simulink subsystem "CLAW_for_QGC_Mission"  (R2024a)
settings: Solver=VariableStepAuto  StartTime=0.0  StopTime=10.0  RelTol=1e-3
undefined symbols (not defined in the file or in its folder): MC_PITCH_P, MC_PITCHRATE_D, MC_PITCHRATE_I, MC_PITCHRATE_P, MC_ROLL_P, MC_ROLLRATE_D, MC_ROLLRATE_I, MC_ROLLRATE_P, MC_YAW_P, MC_YAWRATE_D, MC_YAWRATE_I, MC_YAWRATE_P, MPC_XY_P, MPC_XY_VEL_MAX, MPC_Z_D, MPC_Z_I, MPC_Z_P, MPC_Z_VEL_D_ACC, MPC_Z_VEL_I_ACC, MPC_Z_VEL_MAX_DN, MPC_Z_VEL_MAX_UP, MPC_Z_VEL_P_ACC, pitch, pitch_body, roll, roll_body, thrust_body, timestamp, yaw, yaw_body
libraries: px4lib x25, slpidlib x10, px4uORBlib x4, simulink_extras x4, px4Utilslib x2, sharedutil x1, sharedtransform x1, simulink x1
(part 1 of 2)
settings Model: Creator=user  LastModifiedBy=user

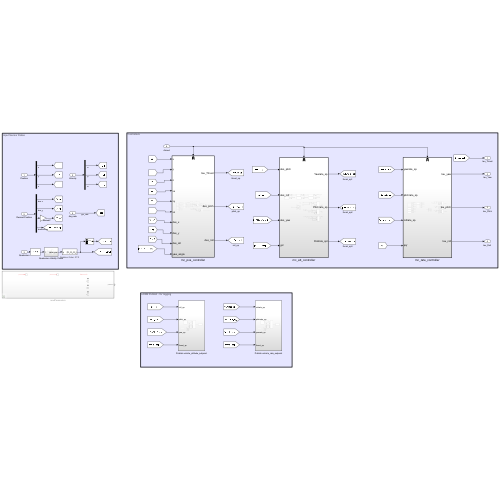
[thumbnail: Simulink's stored preview of the top-level diagram]
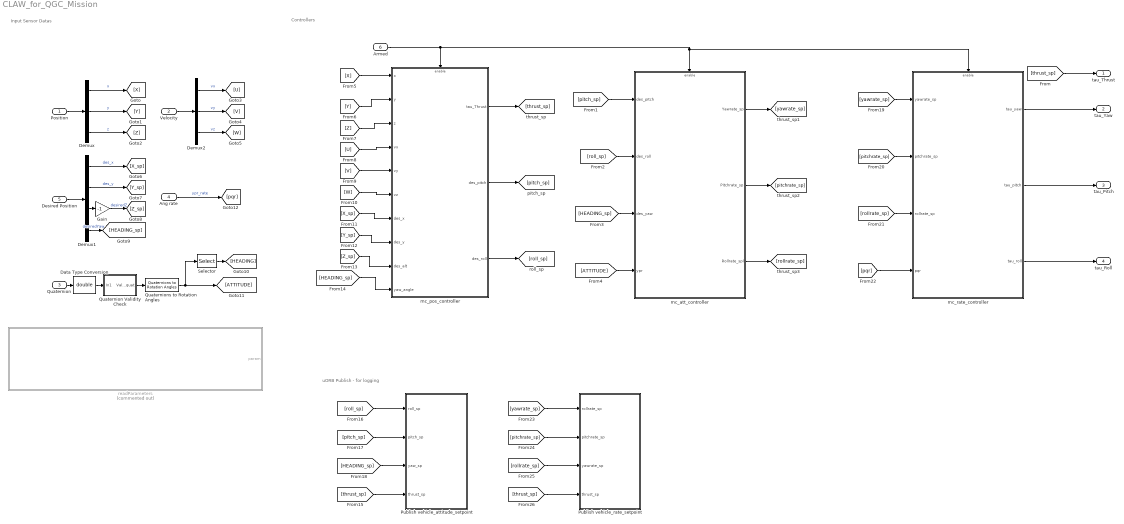
== system CLAW_for_QGC_Mission ==
  note: uORB Publish - for logging
  note: Controllers
  note: Input Sensor Datas
  Position : Inport
  Velocity : Inport  Port=2
  Quaternion : Inport  Port=3
  Ang rate : Inport  Port=4
  Desired Position : Inport  Port=5
  Armed : Inport  Port=6
  Data Type Conversion : DataTypeConversion  OutDataTypeStr=double  SaturateOnIntegerOverflow=off  RndMeth=Floor
  Demux : Demux  Outputs=3
  Demux1 : Demux
  Demux2 : Demux  Outputs=3
  Gain : Gain  Gain=-1
  Publish vehicle_attitude_setpoint : Subsystem
  Publish vehicle_rate_setpoint : Subsystem
  Quaternion Validity Check : Subsystem
  Quaternions to Rotation Angles : sharedtransform/Quaternions to Rotation Angles  rotationOrder=ZYX  aMode=aMode
  Selector : Selector  InputPortWidth=3  IndexOptions=Index vector (dialog)  Indices=[1]  OutputSizes=1
  mc_att_controller : Subsystem
      settings: RTWSystemCode=Nonreusable function  RTWFcnNameOpts=Use subsystem name  RTWFileNameOpts=Use subsystem name
  mc_pos_controller : Subsystem
      settings: RTWSystemCode=Nonreusable function  RTWFcnNameOpts=Use subsystem name  RTWFileNameOpts=Use subsystem name
  mc_rate_controller : Subsystem
      settings: RTWSystemCode=Nonreusable function  RTWFcnNameOpts=Use subsystem name  RTWFileNameOpts=Use subsystem name
  readParameters : Subsystem  Commented=on  TreatAsAtomicUnit=on
  tau_Thrust : Outport
  tau_Yaw : Outport  Port=2
  tau_Pitch : Outport  Port=3
  "tau_Roll " : Outport  Port=4
  wires:
  [Z_sp] -> mc_pos_controller/9(des_alt)
  Armed/1 -> mc_rate_controller/Enable, mc_att_controller/Enable, mc_pos_controller/Enable
  [X_sp] -> mc_pos_controller/7(des_x)
  [pitchrate_sp] -> Publish vehicle_rate_setpoint/2(pitchrate_sp)
  [thrust_sp] -> Publish vehicle_rate_setpoint/4(thrust_sp)
  [V] -> mc_pos_controller/5(vy)
  [pqr] -> mc_rate_controller/4(pqr)
  [HEADING_sp] -> mc_pos_controller/10(yaw_angle)
  [HEADING_sp] -> mc_att_controller/3(des_yaw)
  [U] -> mc_pos_controller/4(vx)
  mc_att_controller/2(Pitchrate_sp) -> [pitchrate_sp]
  [rollrate_sp] -> Publish vehicle_rate_setpoint/3(yawrate_sp)
  [Y] -> mc_pos_controller/2(y)
  mc_att_controller/3(Rollrate_spl) -> [rollrate_sp]
  mc_rate_controller/2(tau_pitch) -> tau_Pitch/1
  [W] -> mc_pos_controller/6(vz)
  [Y_sp] -> mc_pos_controller/8(des_y)
  mc_att_controller/1(Yawrate_sp) -> [yawrate_sp]
  [rollrate_sp] -> mc_rate_controller/3(rollrate_sp)
  [ATTITUDE] -> mc_att_controller/4(ypr)
  [pitch_sp] -> Publish vehicle_attitude_setpoint/2(pitch_sp)
  [thrust_sp] -> Publish vehicle_attitude_setpoint/4(thrust_sp)
  [roll_sp] -> Publish vehicle_attitude_setpoint/1(roll_sp)
  [Z] -> mc_pos_controller/3(z)
  [roll_sp] -> mc_att_controller/2(des_roll)
  Demux2/2 -> [V]  "vy"
  [X] -> mc_pos_controller/1(x)
  [HEADING_sp] -> Publish vehicle_attitude_setpoint/3(yaw_sp)
  [thrust_sp] -> tau_Thrust/1
  [yawrate_sp] -> mc_rate_controller/1(yawrate_sp)
  Quaternion Validity Check/1(Valid quat) -> Quaternions to Rotation Angles/1
  mc_pos_controller/3(des_roll) -> [roll_sp]
  Demux/3 -> [Z]  "z"
  [pitch_sp] -> mc_att_controller/1(des_pitch)
  Quaternions to Rotation Angles/1 -> [ATTITUDE], Selector/1
  mc_rate_controller/1(tau_yaw) -> tau_Yaw/1
  Position/1 -> Demux/1
  Demux/1 -> [X]  "x"
  Demux1/3 -> Gain/1
  Ang rate/1 -> [pqr]  "ypr_rate"
  Demux2/1 -> [U]  "vx"
  Data Type Conversion/1 -> Quaternion Validity Check/1(In1)
  [yawrate_sp] -> Publish vehicle_rate_setpoint/1(rollrate_sp)
  Selector/1 -> [HEADING]
  Gain/1 -> [Z_sp]  "desiredZ"
  Demux1/4 -> [HEADING_sp]  "desiredYaw"
  mc_pos_controller/1(tau_Thrust) -> [thrust_sp]
  Demux1/2 -> [Y_sp]  "des_y"
  Demux2/3 -> [W]  "vz"
  Quaternion/1 -> Data Type Conversion/1
  Demux1/1 -> [X_sp]  "des_x"
  mc_rate_controller/3(tau_roll) -> "tau_Roll "/1
  mc_pos_controller/2(des_pitch) -> [pitch_sp]
  Desired Position/1 -> Demux1/1
  [pitchrate_sp] -> mc_rate_controller/2(pitchrate_sp)
  Velocity/1 -> Demux2/1
  Demux/2 -> [Y]  "y"

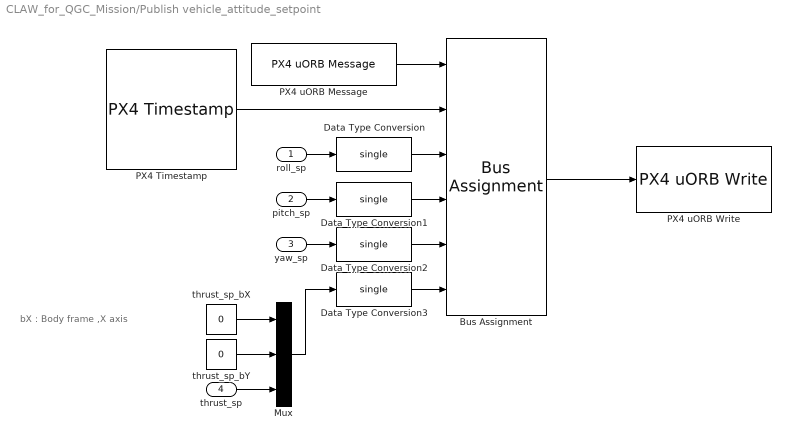
== system CLAW_for_QGC_Mission/Publish vehicle_attitude_setpoint ==
  note: bX : Body frame ,X axis
  roll_sp : Inport
  pitch_sp : Inport  Port=2
  yaw_sp : Inport  Port=3
  thrust_sp : Inport  Port=4
  Bus Assignment : BusAssignment  AssignedSignals=timestamp,roll_body,pitch_body,yaw_body,thrust_body
  Data Type Conversion{,1..3} (4 alike) : DataTypeConversion  OutDataTypeStr=single  SaturateOnIntegerOverflow=off  RndMeth=Floor
  Mux : Mux  Inputs=3
  PX4 Timestamp : px4Utilslib/PX4 Timestamp  SampleTime=-1
  PX4 uORB Message : px4uORBlib/PX4 uORB Message  uORBTopic=VehicleAttitudeSetpoint  SampleTime=-1  selectInstance=vehicle_attitude_setpoint
  PX4 uORB Write : px4uORBlib/PX4 uORB Write  uORBTopic=VehicleAttitudeSetpoint  selectInstance=vehicle_attitude_setpoint  MessageQueueLen=1
  thrust_sp_bX : Constant  Value=0
  thrust_sp_bY : Constant  Value=0
  wires:
  PX4 Timestamp/1 -> Bus Assignment/2
  Bus Assignment/1 -> PX4 uORB Write/1
  PX4 uORB Message/1 -> Bus Assignment/1
  roll_sp/1 -> Data Type Conversion/1
  pitch_sp/1 -> Data Type Conversion1/1
  yaw_sp/1 -> Data Type Conversion2/1
  Data Type Conversion/1 -> Bus Assignment/3
  Data Type Conversion1/1 -> Bus Assignment/4
  Data Type Conversion2/1 -> Bus Assignment/5
  thrust_sp_bX/1 -> Mux/1
  thrust_sp_bY/1 -> Mux/2
  thrust_sp/1 -> Mux/3
  Mux/1 -> Data Type Conversion3/1
  Data Type Conversion3/1 -> Bus Assignment/6

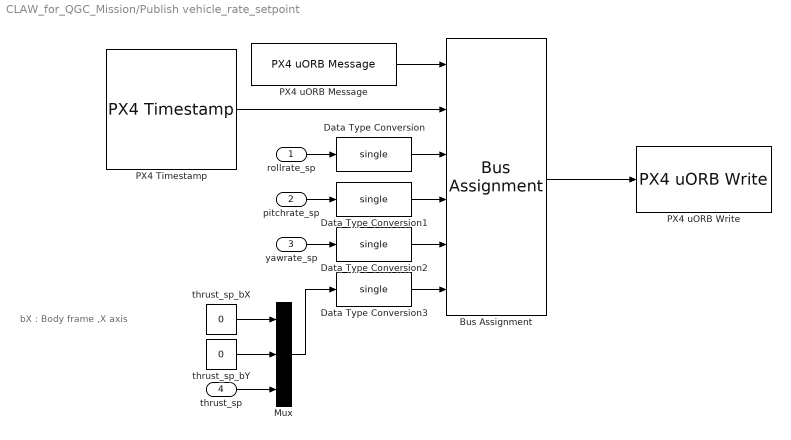
== system CLAW_for_QGC_Mission/Publish vehicle_rate_setpoint ==
  note: bX : Body frame ,X axis
  rollrate_sp : Inport
  pitchrate_sp : Inport  Port=2
  yawrate_sp : Inport  Port=3
  thrust_sp : Inport  Port=4
  Bus Assignment : BusAssignment  AssignedSignals=timestamp,roll,pitch,yaw,thrust_body
  Data Type Conversion{,1..3} (4 alike) : DataTypeConversion  OutDataTypeStr=single  SaturateOnIntegerOverflow=off  RndMeth=Floor
  Mux : Mux  Inputs=3
  PX4 Timestamp : px4Utilslib/PX4 Timestamp  SampleTime=-1
  PX4 uORB Message : px4uORBlib/PX4 uORB Message  uORBTopic=VehicleRatesSetpoint  SampleTime=-1  selectInstance=VehicleRatesSetpoint
  PX4 uORB Write : px4uORBlib/PX4 uORB Write  uORBTopic=VehicleRatesSetpoint  selectInstance=VehicleRatesSetpoint  MessageQueueLen=1
  thrust_sp_bX : Constant  Value=0
  thrust_sp_bY : Constant  Value=0
  wires:
  PX4 Timestamp/1 -> Bus Assignment/2
  Bus Assignment/1 -> PX4 uORB Write/1
  PX4 uORB Message/1 -> Bus Assignment/1
  rollrate_sp/1 -> Data Type Conversion/1
  pitchrate_sp/1 -> Data Type Conversion1/1
  yawrate_sp/1 -> Data Type Conversion2/1
  Data Type Conversion/1 -> Bus Assignment/3
  Data Type Conversion1/1 -> Bus Assignment/4
  Data Type Conversion2/1 -> Bus Assignment/5
  thrust_sp_bX/1 -> Mux/1
  thrust_sp_bY/1 -> Mux/2
  thrust_sp/1 -> Mux/3
  Mux/1 -> Data Type Conversion3/1
  Data Type Conversion3/1 -> Bus Assignment/6

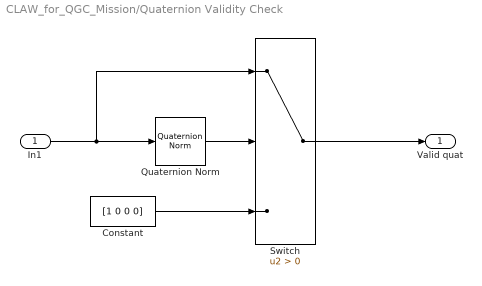
== system CLAW_for_QGC_Mission/Quaternion Validity Check ==
  In1 : Inport
  Constant : Constant  Value=[1 0 0 0]  SampleTime=-1
  Quaternion Norm : sharedutil/Quaternion Norm  aMode=aMode
  Switch : Switch  Criteria=u2 > Threshold  SaturateOnIntegerOverflow=off  InputSameDT=off
  Valid quat : Outport
  wires:
  In1/1 -> Quaternion Norm/1, Switch/1
  Quaternion Norm/1 -> Switch/2
  Switch/1 -> Valid quat/1
  Constant/1 -> Switch/3

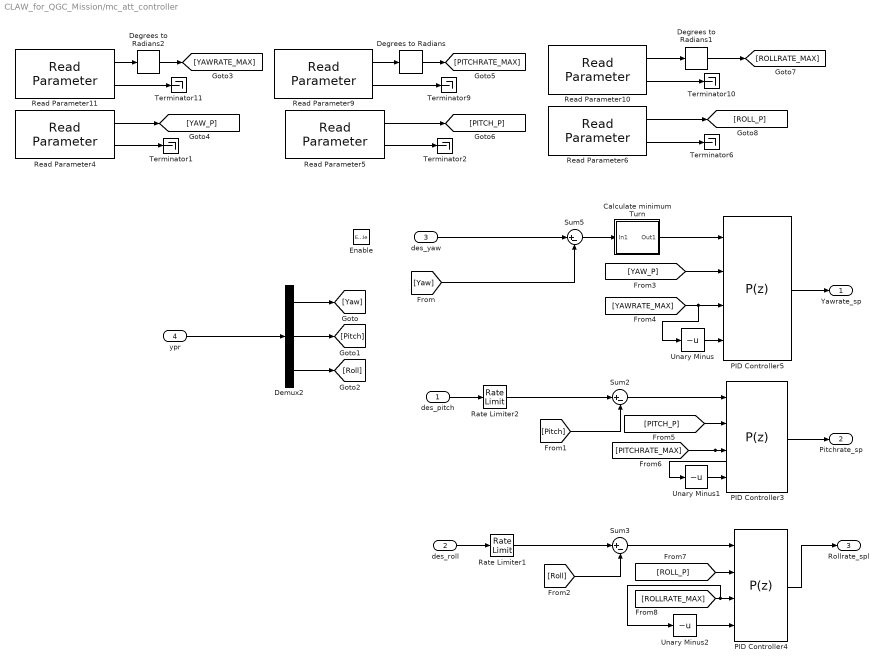
== system CLAW_for_QGC_Mission/mc_att_controller ==
  des_pitch : Inport
  des_roll : Inport  Port=2
  des_yaw : Inport  Port=3
  ypr : Inport  Port=4
  Enable : EnablePort
  Calculate minimum Turn : Subsystem
  Degrees to Radians : simulink_extras/Transformations/Degrees to Radians
  Degrees to Radians1 : simulink_extras/Transformations/Degrees to Radians
  Degrees to Radians2 : simulink_extras/Transformations/Degrees to Radians
  Demux2 : Demux  Outputs=3
  PID Controller3 : slpidlib/PID Controller  Controller=P  Form=Parallel  TimeDomain=Discrete-time  UseExternalTs=off  SampleTime=-1  IntegratorMethod=Forward Euler  FilterMethod=Forward Euler  ControllerParametersSource=external  P=MC_PITCH_P  I=1  UseKiTs=off  D=0  UseExternalDerivativeSource=off  N=100  UseFilter=on  TunerSelectOption=Transfer Function Based (PID Tuner App)  InitialConditionSource=internal  InitialConditionForIntegrator=0  InitialConditionForFilter=0  DifferentiatorICPrevScaledInput=0  ExternalReset=none  TrackingMode=off  Kt=1  LimitOutput=on  SatLimitsSource=external  UpperSaturationLimit=inf  LowerSaturationLimit=-inf  LinearizeAsGain=on  AntiWindupMode=none  Kb=1  LimitIntegrator=off  UpperIntegratorSaturationLimit=inf  LowerIntegratorSaturationLimit=-inf  POutMin=[]  POutMax=[]  IOutMin=[]  IOutMax=[]  DOutMin=[]  DOutMax=[]  NOutMin=[]  NOutMax=[]  SumOutMin=[]  SumOutMax=[]  SaturationOutMin=[]  SaturationOutMax=[]  PParamMin=[]  PParamMax=[]  IParamMin=[]  IParamMax=[]  DParamMin=[]  DParamMax=[]  NParamMin=[]  NParamMax=[]  KbParamMin=[]  KbParamMax=[]  KtParamMin=[]  KtParamMax=[]  KbOutMin=[]  KbOutMax=[]  KtOutMin=[]  KtOutMax=[]  IntegratorOutMin=[]  IntegratorOutMax=[]  FilterOutMin=[]  FilterOutMax=[]  SumI1OutMin=[]  SumI1OutMax=[]  SumI2OutMin=[]  SumI2OutMax=[]  SumI3OutMin=[]  SumI3OutMax=[]  SumI4OutMin=[]  SumI4OutMax=[]  SumDOutMin=[]  SumDOutMax=[]  DifferentiatorOutMin=[]  DifferentiatorOutMax=[]  FilterDiffOutCoefMin=[]  FilterDiffOutCoefMax=[]  ReciprocalOutMin=[]  ReciprocalOutMax=[]  SumDenOutMin=[]  SumDenOutMax=[]  SumNumOutMin=[]  SumNumOutMax=[]  DivideOutMin=[]  DivideOutMax=[]  UdiffTsProdOutMin=[]  UdiffTsProdOutMax=[]  NTsProdOutMin=[]  NTsProdOutMax=[]  UintegralTsProdOutMin=[]  UintegralTsProdOutMax=[]  UngainTsProdOutMin=[]  UngainTsProdOutMax=[]  ClampingZeroOutDataTypeStr=Inherit: Inherit via back propagation  ClampingZeroOutMin=[]  ClampingZeroOutMax=[]  FilterDenConstantOutDataTypeStr=Inherit: Inherit via back propagation  FilterDenConstantOutMin=[]  FilterDenConstantOutMax=[]  PCopyOutDataTypeStr=Inherit: Inherit via back propagation  PCopyOutMin=[]  PCopyOutMax=[]  NCopyOutDataTypeStr=Inherit: Inherit via back propagation  NCopyOutMin=[]  NCopyOutMax=[]  IntegratorContinuousStateAttributes=''  IntegratorStateMustResolveToSignalObject=off  IntegratorRTWStateStorageClass=Auto  FilterContinuousStateAttributes=''  FilterStateMustResolveToSignalObject=off  FilterRTWStateStorageClass=Auto  ParallelPVariant=ExternalParameters  IdealPVariant=Disabled  IVariant=Disabled  DVariant=Disabled  IntegratorVariant=Disabled  SatVariant=External  AWVariant=Disabled  PCopyVariant=Disabled  TRVariant=Disabled  FdbkBlocksVariant=Forward  IdealPFdbkVariant=Disabled  SatFdbkVariant=Disabled  DerivativeFilterVariant=Disabled  NVariant=Disabled  NCopyVariant=Disabled_SignalSpec  FilterICVariant=Disabled  IntegratorICVariant=Disabled  ExternalResetVariant=Disabled  TRSumVariant=Passthrough  SumFdbkVariant=Disabled  SumVariant=Passthrough_P  TsampFilterVariant=InternalTs  TsampNgainVariant=Passthrough  TsampIntegralVariant=Disabled_SignalSpec  ExternalSaturationOutDataTypeStr=Inherit: Same as second input  DerivativeSourceVariant=Disabled
  PID Controller4 : slpidlib/PID Controller  Controller=P  Form=Parallel  TimeDomain=Discrete-time  UseExternalTs=off  SampleTime=-1  IntegratorMethod=Forward Euler  FilterMethod=Forward Euler  ControllerParametersSource=external  P=MC_ROLL_P  I=1  UseKiTs=off  D=0  UseExternalDerivativeSource=off  N=100  UseFilter=on  TunerSelectOption=Transfer Function Based (PID Tuner App)  InitialConditionSource=internal  InitialConditionForIntegrator=0  InitialConditionForFilter=0  DifferentiatorICPrevScaledInput=0  ExternalReset=none  TrackingMode=off  Kt=1  LimitOutput=on  SatLimitsSource=external  UpperSaturationLimit=inf  LowerSaturationLimit=-inf  LinearizeAsGain=on  AntiWindupMode=none  Kb=1  LimitIntegrator=off  UpperIntegratorSaturationLimit=inf  LowerIntegratorSaturationLimit=-inf  POutMin=[]  POutMax=[]  IOutMin=[]  IOutMax=[]  DOutMin=[]  DOutMax=[]  NOutMin=[]  NOutMax=[]  SumOutMin=[]  SumOutMax=[]  SaturationOutMin=[]  SaturationOutMax=[]  PParamMin=[]  PParamMax=[]  IParamMin=[]  IParamMax=[]  DParamMin=[]  DParamMax=[]  NParamMin=[]  NParamMax=[]  KbParamMin=[]  KbParamMax=[]  KtParamMin=[]  KtParamMax=[]  KbOutMin=[]  KbOutMax=[]  KtOutMin=[]  KtOutMax=[]  IntegratorOutMin=[]  IntegratorOutMax=[]  FilterOutMin=[]  FilterOutMax=[]  SumI1OutMin=[]  SumI1OutMax=[]  SumI2OutMin=[]  SumI2OutMax=[]  SumI3OutMin=[]  SumI3OutMax=[]  SumI4OutMin=[]  SumI4OutMax=[]  SumDOutMin=[]  SumDOutMax=[]  DifferentiatorOutMin=[]  DifferentiatorOutMax=[]  FilterDiffOutCoefMin=[]  FilterDiffOutCoefMax=[]  ReciprocalOutMin=[]  ReciprocalOutMax=[]  SumDenOutMin=[]  SumDenOutMax=[]  SumNumOutMin=[]  SumNumOutMax=[]  DivideOutMin=[]  DivideOutMax=[]  UdiffTsProdOutMin=[]  UdiffTsProdOutMax=[]  NTsProdOutMin=[]  NTsProdOutMax=[]  UintegralTsProdOutMin=[]  UintegralTsProdOutMax=[]  UngainTsProdOutMin=[]  UngainTsProdOutMax=[]  ClampingZeroOutDataTypeStr=Inherit: Inherit via back propagation  ClampingZeroOutMin=[]  ClampingZeroOutMax=[]  FilterDenConstantOutDataTypeStr=Inherit: Inherit via back propagation  FilterDenConstantOutMin=[]  FilterDenConstantOutMax=[]  PCopyOutDataTypeStr=Inherit: Inherit via back propagation  PCopyOutMin=[]  PCopyOutMax=[]  NCopyOutDataTypeStr=Inherit: Inherit via back propagation  NCopyOutMin=[]  NCopyOutMax=[]  IntegratorContinuousStateAttributes=''  IntegratorStateMustResolveToSignalObject=off  IntegratorRTWStateStorageClass=Auto  FilterContinuousStateAttributes=''  FilterStateMustResolveToSignalObject=off  FilterRTWStateStorageClass=Auto  ParallelPVariant=ExternalParameters  IdealPVariant=Disabled  IVariant=Disabled  DVariant=Disabled  IntegratorVariant=Disabled  SatVariant=External  AWVariant=Disabled  PCopyVariant=Disabled  TRVariant=Disabled  FdbkBlocksVariant=Forward  IdealPFdbkVariant=Disabled  SatFdbkVariant=Disabled  DerivativeFilterVariant=Disabled  NVariant=Disabled  NCopyVariant=Disabled_SignalSpec  FilterICVariant=Disabled  IntegratorICVariant=Disabled  ExternalResetVariant=Disabled  TRSumVariant=Passthrough  SumFdbkVariant=Disabled  SumVariant=Passthrough_P  TsampFilterVariant=InternalTs  TsampNgainVariant=Passthrough  TsampIntegralVariant=Disabled_SignalSpec  ExternalSaturationOutDataTypeStr=Inherit: Same as second input  DerivativeSourceVariant=Disabled
  PID Controller5 : slpidlib/PID Controller  Controller=P  Form=Parallel  TimeDomain=Discrete-time  UseExternalTs=off  SampleTime=-1  IntegratorMethod=Forward Euler  FilterMethod=Forward Euler  ControllerParametersSource=external  P=MC_YAW_P  I=1  UseKiTs=off  D=0  UseExternalDerivativeSource=off  N=100  UseFilter=on  TunerSelectOption=Transfer Function Based (PID Tuner App)  InitialConditionSource=internal  InitialConditionForIntegrator=0  InitialConditionForFilter=0  DifferentiatorICPrevScaledInput=0  ExternalReset=none  TrackingMode=off  Kt=1  LimitOutput=on  SatLimitsSource=external  UpperSaturationLimit=50*pi/180  LowerSaturationLimit=-50*pi/180  LinearizeAsGain=on  AntiWindupMode=none  Kb=1  LimitIntegrator=off  UpperIntegratorSaturationLimit=inf  LowerIntegratorSaturationLimit=-inf  POutMin=[]  POutMax=[]  IOutMin=[]  IOutMax=[]  DOutMin=[]  DOutMax=[]  NOutMin=[]  NOutMax=[]  SumOutMin=[]  SumOutMax=[]  SaturationOutMin=[]  SaturationOutMax=[]  PParamMin=[]  PParamMax=[]  IParamMin=[]  IParamMax=[]  DParamMin=[]  DParamMax=[]  NParamMin=[]  NParamMax=[]  KbParamMin=[]  KbParamMax=[]  KtParamMin=[]  KtParamMax=[]  KbOutMin=[]  KbOutMax=[]  KtOutMin=[]  KtOutMax=[]  IntegratorOutMin=[]  IntegratorOutMax=[]  FilterOutMin=[]  FilterOutMax=[]  SumI1OutMin=[]  SumI1OutMax=[]  SumI2OutMin=[]  SumI2OutMax=[]  SumI3OutMin=[]  SumI3OutMax=[]  SumI4OutMin=[]  SumI4OutMax=[]  SumDOutMin=[]  SumDOutMax=[]  DifferentiatorOutMin=[]  DifferentiatorOutMax=[]  FilterDiffOutCoefMin=[]  FilterDiffOutCoefMax=[]  ReciprocalOutMin=[]  ReciprocalOutMax=[]  SumDenOutMin=[]  SumDenOutMax=[]  SumNumOutMin=[]  SumNumOutMax=[]  DivideOutMin=[]  DivideOutMax=[]  UdiffTsProdOutMin=[]  UdiffTsProdOutMax=[]  NTsProdOutMin=[]  NTsProdOutMax=[]  UintegralTsProdOutMin=[]  UintegralTsProdOutMax=[]  UngainTsProdOutMin=[]  UngainTsProdOutMax=[]  ClampingZeroOutDataTypeStr=Inherit: Inherit via back propagation  ClampingZeroOutMin=[]  ClampingZeroOutMax=[]  FilterDenConstantOutDataTypeStr=Inherit: Inherit via back propagation  FilterDenConstantOutMin=[]  FilterDenConstantOutMax=[]  PCopyOutDataTypeStr=Inherit: Inherit via back propagation  PCopyOutMin=[]  PCopyOutMax=[]  NCopyOutDataTypeStr=Inherit: Inherit via back propagation  NCopyOutMin=[]  NCopyOutMax=[]  IntegratorContinuousStateAttributes=''  IntegratorStateMustResolveToSignalObject=off  IntegratorRTWStateStorageClass=Auto  FilterContinuousStateAttributes=''  FilterStateMustResolveToSignalObject=off  FilterRTWStateStorageClass=Auto  ParallelPVariant=ExternalParameters  IdealPVariant=Disabled  IVariant=Disabled  DVariant=Disabled  IntegratorVariant=Disabled  SatVariant=External  AWVariant=Disabled  PCopyVariant=Disabled  TRVariant=Disabled  FdbkBlocksVariant=Forward  IdealPFdbkVariant=Disabled  SatFdbkVariant=Disabled  DerivativeFilterVariant=Disabled  NVariant=Disabled  NCopyVariant=Disabled_SignalSpec  FilterICVariant=Disabled  IntegratorICVariant=Disabled  ExternalResetVariant=Disabled  TRSumVariant=Passthrough  SumFdbkVariant=Disabled  SumVariant=Passthrough_P  TsampFilterVariant=InternalTs  TsampNgainVariant=Passthrough  TsampIntegralVariant=Disabled_SignalSpec  ExternalSaturationOutDataTypeStr=Inherit: Same as second input  DerivativeSourceVariant=Disabled
  Rate Limiter1 : RateLimiter  RisingSlewLimit=180*pi/180  FallingSlewLimit=-180*pi/180  SampleTimeMode=inherited
  Rate Limiter2 : RateLimiter  RisingSlewLimit=180*pi/180  FallingSlewLimit=-180*pi/180  SampleTimeMode=inherited
  Read Parameter10 : px4lib/Read Parameter  ParameterName=SL_ROLLRATE_MAX  DataType=FLOAT  SampleTime=-1
  Read Parameter11 : px4lib/Read Parameter  ParameterName=SL_YAWRATE_MAX  DataType=FLOAT  SampleTime=-1
  Read Parameter4 : px4lib/Read Parameter  ParameterName=SL_YAW_P  DataType=FLOAT  SampleTime=-1
  Read Parameter5 : px4lib/Read Parameter  ParameterName=SL_PITCH_P  DataType=FLOAT  SampleTime=-1
  Read Parameter6 : px4lib/Read Parameter  ParameterName=SL_ROLL_P  DataType=FLOAT  SampleTime=-1
  Read Parameter9 : px4lib/Read Parameter  ParameterName=SL_PITCHRATE_MAX  DataType=FLOAT  SampleTime=-1
  Sum2 : Sum  Inputs=|+-
  Sum3 : Sum  Inputs=|+-
  Sum5 : Sum  Inputs=|+-
  Terminator{1..2,6,9..11} (6 alike) : Terminator
  Unary Minus : UnaryMinus
  Unary Minus1 : UnaryMinus
  Unary Minus2 : UnaryMinus
  Yawrate_sp : Outport
  Pitchrate_sp : Outport  Port=2
  Rollrate_spl : Outport  Port=3
  wires:
  Sum2/1 -> PID Controller3/1
  Sum3/1 -> PID Controller4/1
  ypr/1 -> Demux2/1
  Sum5/1 -> Calculate minimum Turn/1(In1)
  Calculate minimum Turn/1(Out1) -> PID Controller5/1
  des_roll/1 -> Rate Limiter1/1
  des_yaw/1 -> Sum5/1
  Rate Limiter1/1 -> Sum3/1
  Rate Limiter2/1 -> Sum2/1
  des_pitch/1 -> Rate Limiter2/1
  PID Controller5/1 -> Yawrate_sp/1
  PID Controller3/1 -> Pitchrate_sp/1
  PID Controller4/1 -> Rollrate_spl/1
  Demux2/1 -> [Yaw]
  Demux2/2 -> [Pitch]
  Demux2/3 -> [Roll]
  [Yaw] -> Sum5/2
  [Pitch] -> Sum2/2
  [Roll] -> Sum3/2
  Read Parameter6/1 -> [ROLL_P]
  Read Parameter4/1 -> [YAW_P]
  Read Parameter5/1 -> [PITCH_P]
  Read Parameter10/2 -> Terminator10/1
  Read Parameter11/1 -> Degrees to Radians2/1
  Read Parameter11/2 -> Terminator11/1
  Read Parameter9/2 -> Terminator9/1
  Read Parameter10/1 -> Degrees to Radians1/1
  Read Parameter9/1 -> Degrees to Radians/1
  Read Parameter4/2 -> Terminator1/1
  Read Parameter5/2 -> Terminator2/1
  Read Parameter6/2 -> Terminator6/1
  [YAW_P] -> PID Controller5/2
  [YAWRATE_MAX] -> Unary Minus/1, PID Controller5/3
  Unary Minus/1 -> PID Controller5/4
  [PITCH_P] -> PID Controller3/2
  [PITCHRATE_MAX] -> Unary Minus1/1, PID Controller3/3
  Unary Minus1/1 -> PID Controller3/4
  [ROLL_P] -> PID Controller4/2
  [ROLLRATE_MAX] -> Unary Minus2/1, PID Controller4/3
  Unary Minus2/1 -> PID Controller4/4
  Degrees to Radians1/1 -> [ROLLRATE_MAX]
  Degrees to Radians/1 -> [PITCHRATE_MAX]
  Degrees to Radians2/1 -> [YAWRATE_MAX]

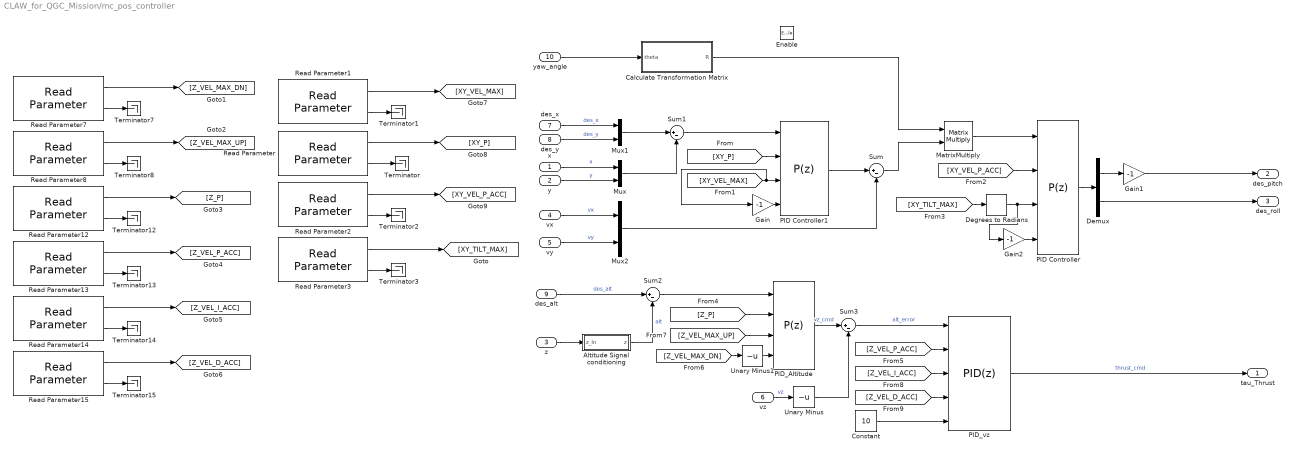
== system CLAW_for_QGC_Mission/mc_pos_controller ==
  x : Inport
  y : Inport  Port=2
  z : Inport  Port=3
  vx : Inport  Port=4
  vy : Inport  Port=5
  vz : Inport  Port=6
  des_x : Inport  Port=7
  des_y : Inport  Port=8
  des_alt : Inport  Port=9
  yaw_angle : Inport  Port=10
  Enable : EnablePort
  Altitude Signal conditioning : Subsystem
  Calculate Transformation Matrix : Subsystem
  Constant : Constant  Value=10
  Degrees to Radians : simulink_extras/Transformations/Degrees to Radians
  Demux : Demux  Outputs=2
  Gain : Gain  Gain=-1
  Gain1 : Gain  Gain=-1
  Gain2 : Gain  Gain=-1
  MatrixMultiply : Product  Multiplication=Matrix(*)
  Mux : Mux  Inputs=2
  Mux1 : Mux  Inputs=2
  Mux2 : Mux  Inputs=2
  PID Controller : slpidlib/PID Controller  Controller=P  Form=Parallel  TimeDomain=Discrete-time  UseExternalTs=off  SampleTime=-1  IntegratorMethod=Forward Euler  FilterMethod=Forward Euler  ControllerParametersSource=external  P=0.3  I=0  UseKiTs=off  D=0  UseExternalDerivativeSource=off  N=20  UseFilter=on  TunerSelectOption=Transfer Function Based (PID Tuner App)  InitialConditionSource=internal  InitialConditionForIntegrator=0  InitialConditionForFilter=0  DifferentiatorICPrevScaledInput=0  ExternalReset=none  TrackingMode=off  Kt=1  LimitOutput=on  SatLimitsSource=external  UpperSaturationLimit=20*pi/180  LowerSaturationLimit=-20*pi/180  LinearizeAsGain=on  AntiWindupMode=clamping  Kb=1  LimitIntegrator=off  UpperIntegratorSaturationLimit=inf  LowerIntegratorSaturationLimit=-inf  POutMin=[]  POutMax=[]  IOutMin=[]  IOutMax=[]  DOutMin=[]  DOutMax=[]  NOutMin=[]  NOutMax=[]  SumOutMin=[]  SumOutMax=[]  SaturationOutMin=[]  SaturationOutMax=[]  PParamMin=[]  PParamMax=[]  IParamMin=[]  IParamMax=[]  DParamMin=[]  DParamMax=[]  NParamMin=[]  NParamMax=[]  KbParamMin=[]  KbParamMax=[]  KtParamMin=[]  KtParamMax=[]  KbOutMin=[]  KbOutMax=[]  KtOutMin=[]  KtOutMax=[]  IntegratorOutMin=[]  IntegratorOutMax=[]  FilterOutMin=[]  FilterOutMax=[]  SumI1OutMin=[]  SumI1OutMax=[]  SumI2OutMin=[]  SumI2OutMax=[]  SumI3OutMin=[]  SumI3OutMax=[]  SumI4OutMin=[]  SumI4OutMax=[]  SumDOutMin=[]  SumDOutMax=[]  DifferentiatorOutMin=[]  DifferentiatorOutMax=[]  FilterDiffOutCoefMin=[]  FilterDiffOutCoefMax=[]  ReciprocalOutMin=[]  ReciprocalOutMax=[]  SumDenOutMin=[]  SumDenOutMax=[]  SumNumOutMin=[]  SumNumOutMax=[]  DivideOutMin=[]  DivideOutMax=[]  UdiffTsProdOutMin=[]  UdiffTsProdOutMax=[]  NTsProdOutMin=[]  NTsProdOutMax=[]  UintegralTsProdOutMin=[]  UintegralTsProdOutMax=[]  UngainTsProdOutMin=[]  UngainTsProdOutMax=[]  ClampingZeroOutDataTypeStr=Inherit: Inherit via back propagation  ClampingZeroOutMin=[]  ClampingZeroOutMax=[]  FilterDenConstantOutDataTypeStr=Inherit: Inherit via back propagation  FilterDenConstantOutMin=[]  FilterDenConstantOutMax=[]  PCopyOutDataTypeStr=Inherit: Inherit via back propagation  PCopyOutMin=[]  PCopyOutMax=[]  NCopyOutDataTypeStr=Inherit: Inherit via back propagation  NCopyOutMin=[]  NCopyOutMax=[]  IntegratorContinuousStateAttributes=''  IntegratorStateMustResolveToSignalObject=off  IntegratorRTWStateStorageClass=Auto  FilterContinuousStateAttributes=''  FilterStateMustResolveToSignalObject=off  FilterRTWStateStorageClass=Auto  ParallelPVariant=ExternalParameters  IdealPVariant=Disabled  IVariant=Disabled  DVariant=Disabled  IntegratorVariant=Disabled  SatVariant=External  AWVariant=Disabled  PCopyVariant=Disabled  TRVariant=Disabled  FdbkBlocksVariant=Forward  IdealPFdbkVariant=Disabled  SatFdbkVariant=Disabled  DerivativeFilterVariant=Disabled  NVariant=Disabled  NCopyVariant=Disabled_SignalSpec  FilterICVariant=Disabled  IntegratorICVariant=Disabled  ExternalResetVariant=Disabled  TRSumVariant=Passthrough  SumFdbkVariant=Disabled  SumVariant=Passthrough_P  TsampFilterVariant=InternalTs  TsampNgainVariant=Passthrough  TsampIntegralVariant=Disabled_SignalSpec  ExternalSaturationOutDataTypeStr=Inherit: Same as second input  DerivativeSourceVariant=Disabled
  PID Controller1 : slpidlib/PID Controller  Controller=P  Form=Parallel  TimeDomain=Discrete-time  UseExternalTs=off  SampleTime=-1  IntegratorMethod=Forward Euler  FilterMethod=Forward Euler  ControllerParametersSource=external  P=MPC_XY_P  I=0  UseKiTs=off  D=0  UseExternalDerivativeSource=off  N=20  UseFilter=on  TunerSelectOption=Transfer Function Based (PID Tuner App)  InitialConditionSource=internal  InitialConditionForIntegrator=0  InitialConditionForFilter=0  DifferentiatorICPrevScaledInput=0  ExternalReset=none  TrackingMode=off  Kt=1  LimitOutput=on  SatLimitsSource=external  UpperSaturationLimit=abs(MPC_XY_VEL_MAX)  LowerSaturationLimit=-abs(MPC_XY_VEL_MAX)  LinearizeAsGain=on  AntiWindupMode=clamping  Kb=1  LimitIntegrator=off  UpperIntegratorSaturationLimit=inf  LowerIntegratorSaturationLimit=-inf  POutMin=[]  POutMax=[]  IOutMin=[]  IOutMax=[]  DOutMin=[]  DOutMax=[]  NOutMin=[]  NOutMax=[]  SumOutMin=[]  SumOutMax=[]  SaturationOutMin=[]  SaturationOutMax=[]  PParamMin=[]  PParamMax=[]  IParamMin=[]  IParamMax=[]  DParamMin=[]  DParamMax=[]  NParamMin=[]  NParamMax=[]  KbParamMin=[]  KbParamMax=[]  KtParamMin=[]  KtParamMax=[]  KbOutMin=[]  KbOutMax=[]  KtOutMin=[]  KtOutMax=[]  IntegratorOutMin=[]  IntegratorOutMax=[]  FilterOutMin=[]  FilterOutMax=[]  SumI1OutMin=[]  SumI1OutMax=[]  SumI2OutMin=[]  SumI2OutMax=[]  SumI3OutMin=[]  SumI3OutMax=[]  SumI4OutMin=[]  SumI4OutMax=[]  SumDOutMin=[]  SumDOutMax=[]  DifferentiatorOutMin=[]  DifferentiatorOutMax=[]  FilterDiffOutCoefMin=[]  FilterDiffOutCoefMax=[]  ReciprocalOutMin=[]  ReciprocalOutMax=[]  SumDenOutMin=[]  SumDenOutMax=[]  SumNumOutMin=[]  SumNumOutMax=[]  DivideOutMin=[]  DivideOutMax=[]  UdiffTsProdOutMin=[]  UdiffTsProdOutMax=[]  NTsProdOutMin=[]  NTsProdOutMax=[]  UintegralTsProdOutMin=[]  UintegralTsProdOutMax=[]  UngainTsProdOutMin=[]  UngainTsProdOutMax=[]  ClampingZeroOutDataTypeStr=Inherit: Inherit via back propagation  ClampingZeroOutMin=[]  ClampingZeroOutMax=[]  FilterDenConstantOutDataTypeStr=Inherit: Inherit via back propagation  FilterDenConstantOutMin=[]  FilterDenConstantOutMax=[]  PCopyOutDataTypeStr=Inherit: Inherit via back propagation  PCopyOutMin=[]  PCopyOutMax=[]  NCopyOutDataTypeStr=Inherit: Inherit via back propagation  NCopyOutMin=[]  NCopyOutMax=[]  IntegratorContinuousStateAttributes=''  IntegratorStateMustResolveToSignalObject=off  IntegratorRTWStateStorageClass=Auto  FilterContinuousStateAttributes=''  FilterStateMustResolveToSignalObject=off  FilterRTWStateStorageClass=Auto  ParallelPVariant=ExternalParameters  IdealPVariant=Disabled  IVariant=Disabled  DVariant=Disabled  IntegratorVariant=Disabled  SatVariant=External  AWVariant=Disabled  PCopyVariant=Disabled  TRVariant=Disabled  FdbkBlocksVariant=Forward  IdealPFdbkVariant=Disabled  SatFdbkVariant=Disabled  DerivativeFilterVariant=Disabled  NVariant=Disabled  NCopyVariant=Disabled_SignalSpec  FilterICVariant=Disabled  IntegratorICVariant=Disabled  ExternalResetVariant=Disabled  TRSumVariant=Passthrough  SumFdbkVariant=Disabled  SumVariant=Passthrough_P  TsampFilterVariant=InternalTs  TsampNgainVariant=Passthrough  TsampIntegralVariant=Disabled_SignalSpec  ExternalSaturationOutDataTypeStr=Inherit: Same as second input  DerivativeSourceVariant=Disabled
  PID_Altitude : slpidlib/PID Controller  Controller=P  Form=Parallel  TimeDomain=Discrete-time  UseExternalTs=off  SampleTime=-1  IntegratorMethod=Backward Euler  FilterMethod=Forward Euler  ControllerParametersSource=external  P=MPC_Z_P  I=MPC_Z_I  UseKiTs=off  D=MPC_Z_D  UseExternalDerivativeSource=off  N=10  UseFilter=on  TunerSelectOption=Transfer Function Based (PID Tuner App)  InitialConditionSource=internal  InitialConditionForIntegrator=0  InitialConditionForFilter=0  DifferentiatorICPrevScaledInput=0  ExternalReset=none  TrackingMode=off  Kt=1  LimitOutput=on  SatLimitsSource=external  UpperSaturationLimit=MPC_Z_VEL_MAX_UP  LowerSaturationLimit=-abs(MPC_Z_VEL_MAX_DN)  LinearizeAsGain=off  AntiWindupMode=clamping  Kb=1  LimitIntegrator=off  UpperIntegratorSaturationLimit=inf  LowerIntegratorSaturationLimit=-inf  POutMin=[]  POutMax=[]  IOutMin=[]  IOutMax=[]  DOutMin=[]  DOutMax=[]  NOutMin=[]  NOutMax=[]  SumOutMin=[]  SumOutMax=[]  SaturationOutMin=[]  SaturationOutMax=[]  PParamMin=[]  PParamMax=[]  IParamMin=[]  IParamMax=[]  DParamMin=[]  DParamMax=[]  NParamMin=[]  NParamMax=[]  KbParamMin=[]  KbParamMax=[]  KtParamMin=[]  KtParamMax=[]  KbOutMin=[]  KbOutMax=[]  KtOutMin=[]  KtOutMax=[]  IntegratorOutMin=[]  IntegratorOutMax=[]  FilterOutMin=[]  FilterOutMax=[]  SumI1OutMin=[]  SumI1OutMax=[]  SumI2OutMin=[]  SumI2OutMax=[]  SumI3OutMin=[]  SumI3OutMax=[]  SumI4OutMin=[]  SumI4OutMax=[]  SumDOutMin=[]  SumDOutMax=[]  DifferentiatorOutMin=[]  DifferentiatorOutMax=[]  FilterDiffOutCoefMin=[]  FilterDiffOutCoefMax=[]  ReciprocalOutMin=[]  ReciprocalOutMax=[]  SumDenOutMin=[]  SumDenOutMax=[]  SumNumOutMin=[]  SumNumOutMax=[]  DivideOutMin=[]  DivideOutMax=[]  UdiffTsProdOutMin=[]  UdiffTsProdOutMax=[]  NTsProdOutMin=[]  NTsProdOutMax=[]  UintegralTsProdOutMin=[]  UintegralTsProdOutMax=[]  UngainTsProdOutMin=[]  UngainTsProdOutMax=[]  ClampingZeroOutDataTypeStr=Inherit: Inherit via back propagation  ClampingZeroOutMin=[]  ClampingZeroOutMax=[]  FilterDenConstantOutDataTypeStr=Inherit: Inherit via back propagation  FilterDenConstantOutMin=[]  FilterDenConstantOutMax=[]  PCopyOutDataTypeStr=Inherit: Inherit via back propagation  PCopyOutMin=[]  PCopyOutMax=[]  NCopyOutDataTypeStr=Inherit: Inherit via back propagation  NCopyOutMin=[]  NCopyOutMax=[]  IntegratorContinuousStateAttributes=''  IntegratorStateMustResolveToSignalObject=off  IntegratorRTWStateStorageClass=Auto  FilterContinuousStateAttributes=''  FilterStateMustResolveToSignalObject=off  FilterRTWStateStorageClass=Auto  ParallelPVariant=ExternalParameters  IdealPVariant=Disabled  IVariant=Disabled  DVariant=Disabled  IntegratorVariant=Disabled  SatVariant=External  AWVariant=Disabled  PCopyVariant=Disabled  TRVariant=Disabled  FdbkBlocksVariant=Forward  IdealPFdbkVariant=Disabled  SatFdbkVariant=Disabled  DerivativeFilterVariant=Disabled  NVariant=Disabled  NCopyVariant=Disabled_SignalSpec  FilterICVariant=Disabled  IntegratorICVariant=Disabled  ExternalResetVariant=Disabled  TRSumVariant=Passthrough  SumFdbkVariant=Disabled  SumVariant=Passthrough_P  TsampFilterVariant=InternalTs  TsampNgainVariant=Passthrough  TsampIntegralVariant=Disabled_SignalSpec  ExternalSaturationOutDataTypeStr=Inherit: Same as second input  DerivativeSourceVariant=Disabled
  PID_vz : slpidlib/PID Controller  Controller=PID  Form=Parallel  TimeDomain=Discrete-time  UseExternalTs=off  SampleTime=-1  IntegratorMethod=Backward Euler  FilterMethod=Forward Euler  ControllerParametersSource=external  P=MPC_Z_VEL_P_ACC  I=MPC_Z_VEL_I_ACC  UseKiTs=off  D=MPC_Z_VEL_D_ACC  UseExternalDerivativeSource=off  N=10  UseFilter=on  TunerSelectOption=Transfer Function Based (PID Tuner App)  InitialConditionSource=internal  InitialConditionForIntegrator=0  InitialConditionForFilter=0  DifferentiatorICPrevScaledInput=0  ExternalReset=none  TrackingMode=off  Kt=1  LimitOutput=on  SatLimitsSource=internal  UpperSaturationLimit=1  LowerSaturationLimit=0  LinearizeAsGain=off  AntiWindupMode=clamping  Kb=1  LimitIntegrator=off  UpperIntegratorSaturationLimit=inf  LowerIntegratorSaturationLimit=-inf  POutMin=[]  POutMax=[]  IOutMin=[]  IOutMax=[]  DOutMin=[]  DOutMax=[]  NOutMin=[]  NOutMax=[]  SumOutMin=[]  SumOutMax=[]  SaturationOutMin=[]  SaturationOutMax=[]  PParamMin=[]  PParamMax=[]  IParamMin=[]  IParamMax=[]  DParamMin=[]  DParamMax=[]  NParamMin=[]  NParamMax=[]  KbParamMin=[]  KbParamMax=[]  KtParamMin=[]  KtParamMax=[]  KbOutMin=[]  KbOutMax=[]  KtOutMin=[]  KtOutMax=[]  IntegratorOutMin=[]  IntegratorOutMax=[]  FilterOutMin=[]  FilterOutMax=[]  SumI1OutMin=[]  SumI1OutMax=[]  SumI2OutMin=[]  SumI2OutMax=[]  SumI3OutMin=[]  SumI3OutMax=[]  SumI4OutMin=[]  SumI4OutMax=[]  SumDOutMin=[]  SumDOutMax=[]  DifferentiatorOutMin=[]  DifferentiatorOutMax=[]  FilterDiffOutCoefMin=[]  FilterDiffOutCoefMax=[]  ReciprocalOutMin=[]  ReciprocalOutMax=[]  SumDenOutMin=[]  SumDenOutMax=[]  SumNumOutMin=[]  SumNumOutMax=[]  DivideOutMin=[]  DivideOutMax=[]  UdiffTsProdOutMin=[]  UdiffTsProdOutMax=[]  NTsProdOutMin=[]  NTsProdOutMax=[]  UintegralTsProdOutMin=[]  UintegralTsProdOutMax=[]  UngainTsProdOutMin=[]  UngainTsProdOutMax=[]  ClampingZeroOutDataTypeStr=Inherit: Inherit via back propagation  ClampingZeroOutMin=[]  ClampingZeroOutMax=[]  FilterDenConstantOutDataTypeStr=Inherit: Inherit via back propagation  FilterDenConstantOutMin=[]  FilterDenConstantOutMax=[]  PCopyOutDataTypeStr=Inherit: Inherit via back propagation  PCopyOutMin=[]  PCopyOutMax=[]  NCopyOutDataTypeStr=Inherit: Inherit via back propagation  NCopyOutMin=[]  NCopyOutMax=[]  IntegratorContinuousStateAttributes=''  IntegratorStateMustResolveToSignalObject=off  IntegratorRTWStateStorageClass=Auto  FilterContinuousStateAttributes=''  FilterStateMustResolveToSignalObject=off  FilterRTWStateStorageClass=Auto  ParallelPVariant=ExternalParameters  IdealPVariant=Disabled  IVariant=ExternalParameters  DVariant=ExternalParameters  IntegratorVariant=Discrete  SatVariant=Enabled  AWVariant=DiscClampingParallel  PCopyVariant=Disabled  TRVariant=Disabled  FdbkBlocksVariant=Feedback  IdealPFdbkVariant=Passthrough  SatFdbkVariant=Passthrough  DerivativeFilterVariant=ForwardEulerFilter  NVariant=ExternalParameters  NCopyVariant=Disabled  FilterICVariant=InternalICsFilter  IntegratorICVariant=InternalICs  ExternalResetVariant=Disabled  TRSumVariant=Passthrough  SumFdbkVariant=Enabled  SumVariant=Sum_PID  TsampFilterVariant=InternalTs  TsampNgainVariant=Passthrough  TsampIntegralVariant=Disabled_SignalSpec  ExternalSaturationOutDataTypeStr=Inherit: Same as second input  DerivativeSourceVariant=ErrorSignal
  Read Parameter : px4lib/Read Parameter  ParameterName=SL_XY_P  DataType=FLOAT  SampleTime=-1
  Read Parameter1 : px4lib/Read Parameter  ParameterName=SL_XY_VEL_MAX  DataType=FLOAT  SampleTime=-1
  Read Parameter12 : px4lib/Read Parameter  ParameterName=SL_Z_P  DataType=FLOAT  SampleTime=-1
  Read Parameter13 : px4lib/Read Parameter  ParameterName=SL_Z_VEL_P_ACC  DataType=FLOAT  SampleTime=-1
  Read Parameter14 : px4lib/Read Parameter  ParameterName=SL_Z_VEL_I_ACC  DataType=FLOAT  SampleTime=-1
  Read Parameter15 : px4lib/Read Parameter  ParameterName=SL_Z_VEL_D_ACC  DataType=FLOAT  SampleTime=-1
  Read Parameter2 : px4lib/Read Parameter  ParameterName=SL_XY_VEL_P_ACC  DataType=FLOAT  SampleTime=-1
  Read Parameter3 : px4lib/Read Parameter  ParameterName=SL_XY_TILT_MAX  DataType=FLOAT  SampleTime=-1
  Read Parameter7 : px4lib/Read Parameter  ParameterName=SL_Z_VEL_MAX_DN  DataType=FLOAT  SampleTime=-1
  Read Parameter8 : px4lib/Read Parameter  ParameterName=SL_Z_VEL_MAX_UP  DataType=FLOAT  SampleTime=-1
  Sum{,1..3} (4 alike) : Sum  Inputs=|+-
  Terminator{,1..3,7..8,12..15} (10 alike) : Terminator
  Unary Minus : UnaryMinus
  Unary Minus1 : UnaryMinus
  tau_Thrust : Outport
  des_pitch : Outport  Port=2
  des_roll : Outport  Port=3
  wires:
  des_alt/1 -> Sum2/1  "des_alt"
  Calculate Transformation Matrix/1(R) -> MatrixMultiply/1
  yaw_angle/1 -> Calculate Transformation Matrix/1(theta)
  Altitude Signal conditioning/1(z) -> Sum2/2  "alt"
  PID_Altitude/1 -> Sum3/1  "vz_cmd"
  vz/1 -> Unary Minus/1  "vz"
  PID_vz/1 -> tau_Thrust/1  "thrust_cmd"
  vx/1 -> Mux2/1  "vx"
  vy/1 -> Mux2/2  "vy"
  Sum2/1 -> PID_Altitude/1
  z/1 -> Altitude Signal conditioning/1(z_In)
  PID Controller/1 -> Demux/1
  Demux/1 -> Gain1/1
  x/1 -> Mux/1  "x"
  y/1 -> Mux/2  "y"
  Demux/2 -> des_roll/1
  Sum/1 -> MatrixMultiply/2
  Mux/1 -> Sum1/2
  Sum1/1 -> PID Controller1/1
  Unary Minus/1 -> Sum3/2
  Sum3/1 -> PID_vz/1  "alt_error"
  des_x/1 -> Mux1/1  "des_x"
  des_y/1 -> Mux1/2  "des_y"
  MatrixMultiply/1 -> PID Controller/1
  PID Controller1/1 -> Sum/1
  Mux1/1 -> Sum1/1
  Gain1/1 -> des_pitch/1
  Mux2/1 -> Sum/2
  Read Parameter14/2 -> Terminator14/1
  Read Parameter12/2 -> Terminator12/1
  Read Parameter14/1 -> [Z_VEL_I_ACC]
  Read Parameter/1 -> [XY_P]
  Read Parameter13/1 -> [Z_VEL_P_ACC]
  Read Parameter8/1 -> [Z_VEL_MAX_UP]
  Read Parameter3/2 -> Terminator3/1
  Read Parameter12/1 -> [Z_P]
  Read Parameter8/2 -> Terminator8/1
  Read Parameter7/2 -> Terminator7/1
  Read Parameter1/1 -> [XY_VEL_MAX]
  Read Parameter2/1 -> [XY_VEL_P_ACC]
  Read Parameter2/2 -> Terminator2/1
  Read Parameter15/1 -> [Z_VEL_D_ACC]
  Read Parameter1/2 -> Terminator1/1
  Read Parameter3/1 -> [XY_TILT_MAX]
  Read Parameter13/2 -> Terminator13/1
  Read Parameter/2 -> Terminator/1
  Read Parameter15/2 -> Terminator15/1
  [XY_P] -> PID Controller1/2
  [XY_VEL_MAX] -> PID Controller1/3, Gain/1
  Gain/1 -> PID Controller1/4
  [XY_VEL_P_ACC] -> PID Controller/2
  [XY_TILT_MAX] -> Degrees to Radians/1
  Degrees to Radians/1 -> Gain2/1, PID Controller/3
  Gain2/1 -> PID Controller/4
  Read Parameter7/1 -> [Z_VEL_MAX_DN]
  [Z_P] -> PID_Altitude/2
  [Z_VEL_MAX_UP] -> PID_Altitude/3
  [Z_VEL_P_ACC] -> PID_vz/2
  [Z_VEL_I_ACC] -> PID_vz/3
  [Z_VEL_D_ACC] -> PID_vz/4
  Constant/1 -> PID_vz/5
  [Z_VEL_MAX_DN] -> Unary Minus1/1
  Unary Minus1/1 -> PID_Altitude/4
